simulink model "Simulador_lineal"  (R2023a)
settings: Solver=FixedStepAuto  StartTime=0.0  StopTime=70  FixedStep=Ts  RelTol=1e-3
undefined symbols (not defined in the file): FC, NP, Ts, TsMot, TsPos, TsRef, TsSenF, TsVel, uo
libraries: simulink x1
settings Model: Creator=rrico  LastModifiedBy=jarico
settings OptimizationCC: ReuseModelBlockBuffer=off

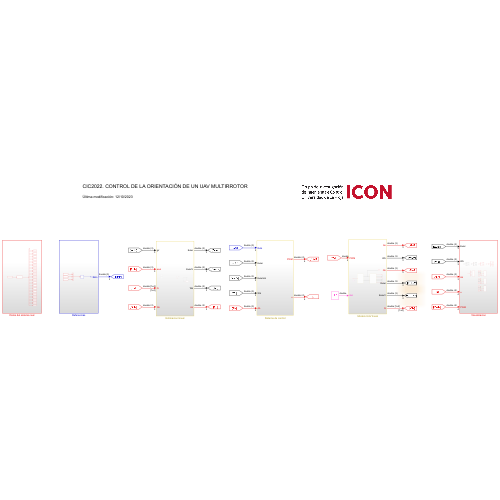
[thumbnail: Simulink's stored preview of the top-level diagram]
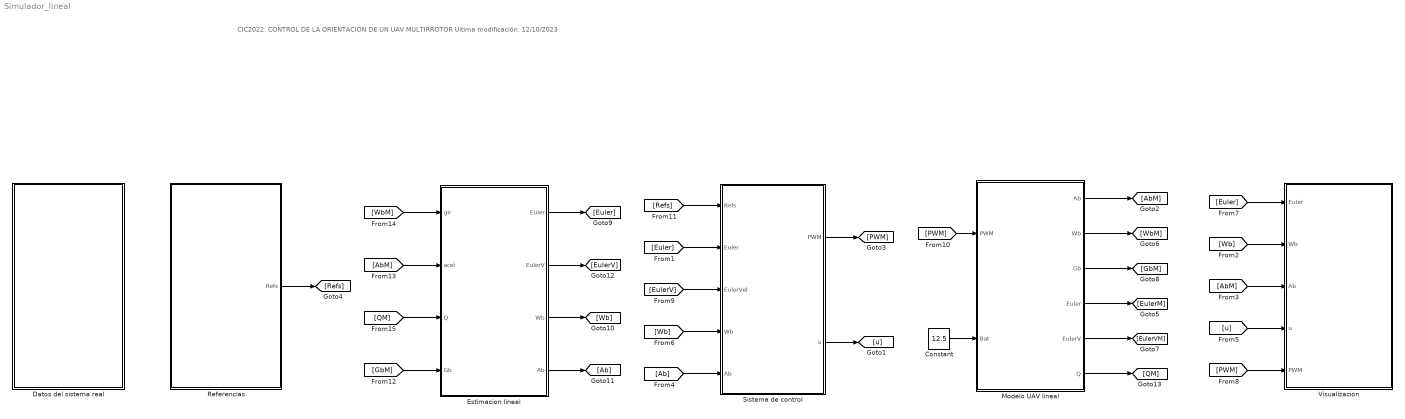
== system Simulador_lineal ==
  note: CIC2022. CONTROL DE LA ORIENTACIÓN DE UN UAV MULTIRROTOR
      |
      | Última modificación: 12/10/2023
  Constant : Constant  Value=12.5
  Datos del sistema real : Subsystem
  Estimacion lineal : Subsystem
  Modelo UAV lineal : Subsystem
  Referencias : Subsystem
  Sistema de control : Subsystem
  Visualizacion : Subsystem
  wires:
  Referencias/1(Refs) -> [Refs]
  [Wb] -> Visualizacion/2(Wb)
  [AbM] -> Visualizacion/3(Ab)
  [PWM] -> Visualizacion/5(PWM)
  [u] -> Visualizacion/4(u)
  Constant/1 -> Modelo UAV lineal/2(Bat)
  Sistema de control/1(PWM) -> [PWM]
  [PWM] -> Modelo UAV lineal/1(PWM)
  Modelo UAV lineal/2(Wb) -> [WbM]
  Modelo UAV lineal/1(Ab) -> [AbM]
  [Refs] -> Sistema de control/1(Refs)
  [Wb] -> Sistema de control/4(Wb)
  Sistema de control/2(u) -> [u]
  [Euler] -> Sistema de control/2(Euler)
  Modelo UAV lineal/4(Euler) -> [EulerM]
  [Euler] -> Visualizacion/1(Euler)
  [Ab] -> Sistema de control/5(Ab)
  Modelo UAV lineal/5(EulerV) -> [EulerVM]
  [EulerV] -> Sistema de control/3(EulerVel)
  Modelo UAV lineal/3(Gb) -> [GbM]
  Estimacion lineal/1(Euler) -> [Euler]
  Estimacion lineal/3(Wb) -> [Wb]
  Estimacion lineal/4(Ab) -> [Ab]
  Estimacion lineal/2(EulerV) -> [EulerV]
  Modelo UAV lineal/6(Q) -> [QM]
  [GbM] -> Estimacion lineal/4(Gb)
  [QM] -> Estimacion lineal/3(Q)
  [AbM] -> Estimacion lineal/2(acel)
  [WbM] -> Estimacion lineal/1(gir)

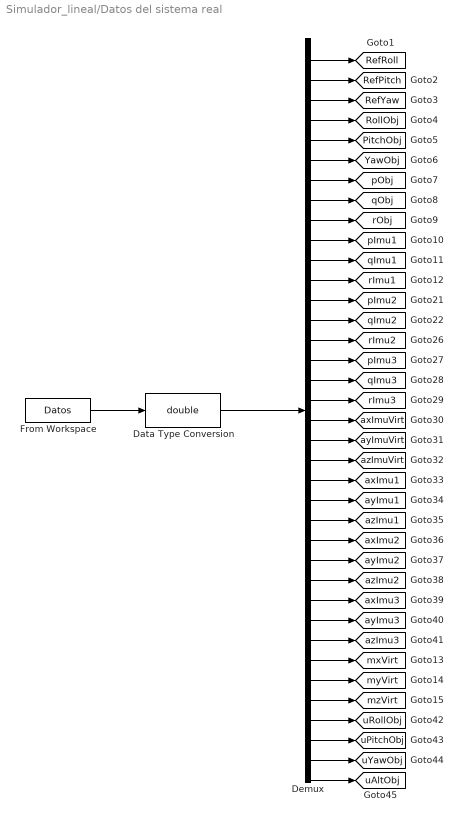
== system Simulador_lineal/Datos del sistema real ==
  Data Type Conversion : DataTypeConversion  OutDataTypeStr=double  SaturateOnIntegerOverflow=off  RndMeth=Floor
  Demux : Demux  Outputs=38
  From Workspace : FromWorkspace  VariableName=Datos  SampleTime=Ts
  tag scope: PitchObj=global, RefPitch=global, RefRoll=global, RefYaw=global, RollObj=global, YawObj=global, axImu1=global, axImu2=global, axImu3=global, axImuVirt=global, ayImu1=global, ayImu2=global, ayImu3=global, ayImuVirt=global, azImu1=global, azImu2=global, azImu3=global, azImuVirt=global, mxVirt=global, myVirt=global, mzVirt=global, pImu1=global, pImu2=global, pImu3=global, pObj=global, qImu1=global, qImu2=global, qImu3=global, qObj=global, rImu1=global, rImu2=global, rImu3=global, rObj=global, uAltObj=global, uPitchObj=global, uRollObj=global, uYawObj=global
  wires:
  Demux/31 -> [azImu3]
  Demux/7 -> [YawObj]
  Demux/17 -> [pImu3]
  Demux/25 -> [azImu1]
  Demux/27 -> [ayImu2]
  Demux/16 -> [rImu2]
  Demux/15 -> [qImu2]
  Demux/30 -> [ayImu3]
  Demux/21 -> [ayImuVirt]
  Demux/10 -> [rObj]
  Demux/2 -> [RefRoll]
  Demux/24 -> [ayImu1]
  Demux/5 -> [RollObj]
  Demux/29 -> [axImu3]
  Demux/8 -> [pObj]
  Demux/28 -> [azImu2]
  Demux/18 -> [qImu3]
  Demux/6 -> [PitchObj]
  Demux/19 -> [rImu3]
  Data Type Conversion/1 -> Demux/1
  Demux/4 -> [RefYaw]
  Demux/22 -> [azImuVirt]
  From Workspace/1 -> Data Type Conversion/1
  Demux/23 -> [axImu1]
  Demux/9 -> [qObj]
  Demux/13 -> [rImu1]
  Demux/3 -> [RefPitch]
  Demux/26 -> [axImu2]
  Demux/11 -> [pImu1]
  Demux/14 -> [pImu2]
  Demux/38 -> [uAltObj]
  Demux/37 -> [uYawObj]
  Demux/36 -> [uPitchObj]
  Demux/35 -> [uRollObj]
  Demux/32 -> [mxVirt]
  Demux/33 -> [myVirt]
  Demux/34 -> [mzVirt]
  Demux/20 -> [axImuVirt]
  Demux/12 -> [qImu1]

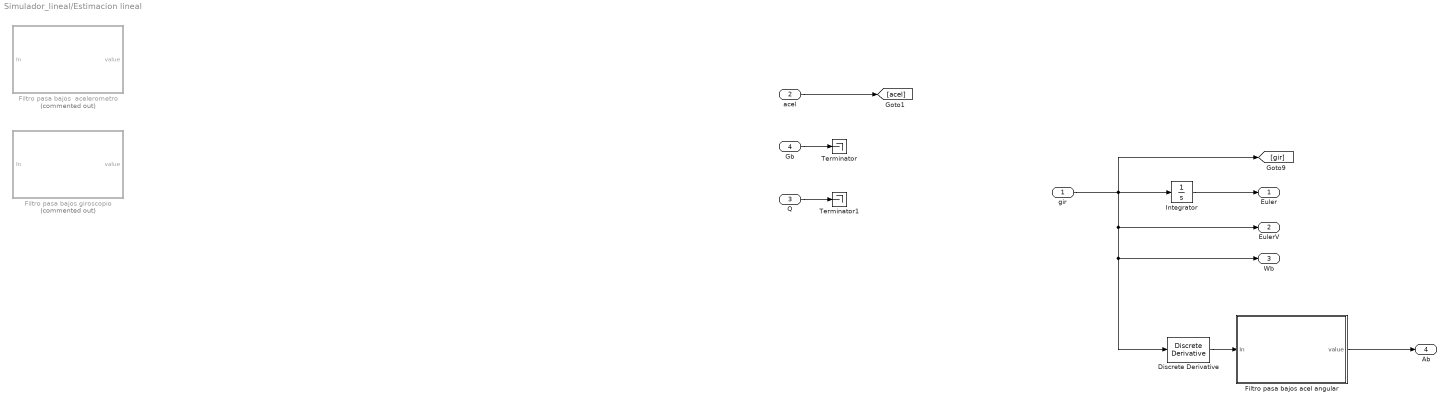
== system Simulador_lineal/Estimacion lineal ==
  gir : Inport
  acel : Inport  Port=2
  Q : Inport  Port=3
  Gb : Inport  Port=4
  Discrete Derivative : simulink/Discrete/Discrete Derivative  gainval=1.0  ICPrevScaledInput=0.0  OutMin=[]  OutMax=[]  OutDataType=fixdt(1, 16)  OutScaling=2^-10  DoSatur=off
  Filtro pasa bajos  acelerometro : Subsystem  Commented=on  TreatAsAtomicUnit=on  SystemSampleTime=TsSenF  mask{P=NP, Fc=FC, TsF=TsSenF}
      mask prompts: P "Polos"; Fc "Frecuencia de corte"; TsF "Tiempo de muestreo"
      mask DialogControl ParameterGroup1 Prompt: Parameters
  Filtro pasa bajos acel angular : Subsystem  TreatAsAtomicUnit=on  SystemSampleTime=TsVel  mask{P=2, Fc=30, TsF=TsSenF}
      mask prompts: P "Polos"; Fc "Frecuencia de corte"; TsF "Tiempo de muestreo"
      mask DialogControl ParameterGroup1 Prompt: Parameters
  Filtro pasa bajos giroscopio : Subsystem  Commented=on  TreatAsAtomicUnit=on  SystemSampleTime=TsSenF  mask{P=NP, Fc=FC, TsF=TsSenF}
      mask prompts: P "Polos"; Fc "Frecuencia de corte"; TsF "Tiempo de muestreo"
      mask DialogControl ParameterGroup1 Prompt: Parameters
  Integrator : Integrator
  Terminator : Terminator
  Terminator1 : Terminator
  Euler : Outport
  EulerV : Outport  Port=2
  Wb : Outport  Port=3
  Ab : Outport  Port=4
  wires:
  Discrete Derivative/1 -> Filtro pasa bajos acel angular/1(In)
  Filtro pasa bajos acel angular/1(value) -> Ab/1
  Gb/1 -> Terminator/1
  Q/1 -> Terminator1/1
  acel/1 -> [acel]
  gir/1 -> [gir], Integrator/1, Discrete Derivative/1, Wb/1, EulerV/1
  Integrator/1 -> Euler/1

== system Simulador_lineal/Modelo UAV lineal ==
  PWM : Inport
  Bat : Inport  Port=2
  Dinamica UAV : Subsystem  mask{Mo=[0 0 0], B=[0.002 0.005 0.005]*0, F=[0.025 0.006 0.006]*0, I=[0.0014 0.025 0.0549], Im=0.0005, dM=0, M=0.2472, Dr=0.09, Dp=0.0675, Y=off, Mq=on}
      mask prompts: Mo "Par inicial"; B "Rozamiento viscoso"; F "Rozamiento estático"; I "Inercia"; Im "Inercia del rotor"; dM "Distancia del centro de masas"; M "Masa"; Dr "Distancia de los rotores a roll"; Dp "Distancia de los rotores a pitch"; Y "Habilitacion yaw"; Mq "Modelo de maqueta"
      mask DialogControl DescTextVar Prompt: Modelo dinámico del UAV
      mask DialogControl Parameter1 Prompt: Rozamientos y pares adicionales
      mask DialogControl Parameter2 Prompt: Parámetros físicos
      mask DialogControl Parameter3 Prompt: Selectores
  Scope : Scope
  Sistema de propulsion : Subsystem  mask{k=9.0893, kd=0, Tau=0.05}
      mask prompts: k "Ganancia en thrust"; kd "Ganancia en drag"; Tau "Dinamica"
      mask DialogControl ParameterGroupVar1 Prompt: Estatica del motor
      mask DialogControl ParameterGroupVar2 Prompt: Dinamica del motor
  Terminator : Terminator
  Ab : Outport
  Wb : Outport  Port=2
  Gb : Outport  Port=3
  Euler : Outport  Port=4
  EulerV : Outport  Port=5
  Q : Outport  Port=6
  wires:
  Dinamica UAV/6(Q) -> Q/1
  Dinamica UAV/5(EulerV) -> EulerV/1
  Dinamica UAV/4(Euler) -> Euler/1
  Dinamica UAV/1(Ab) -> Ab/1
  Sistema de propulsion/1(T) -> Scope/1, Dinamica UAV/1(T)
  Dinamica UAV/2(Wb) -> Wb/1
  Sistema de propulsion/2(D) -> Dinamica UAV/2(Delta)
  Dinamica UAV/3(Gb) -> Gb/1
  PWM/1 -> Sistema de propulsion/1(PWM)
  Bat/1 -> Terminator/1

== system Simulador_lineal/Referencias ==
  Mux17 : Mux  Inputs=3
  Zero-Order Hold : ZeroOrderHold  SampleTime=TsRef
  Refs : Outport  VectorParamsAs1DForOutWhenUnconnected=off
  wires:
  Zero-Order Hold/1 -> Refs/1
  [RefYaw] -> Mux17/3
  [RefPitch] -> Mux17/2
  [RefRoll] -> Mux17/1
  Mux17/1 -> Zero-Order Hold/1

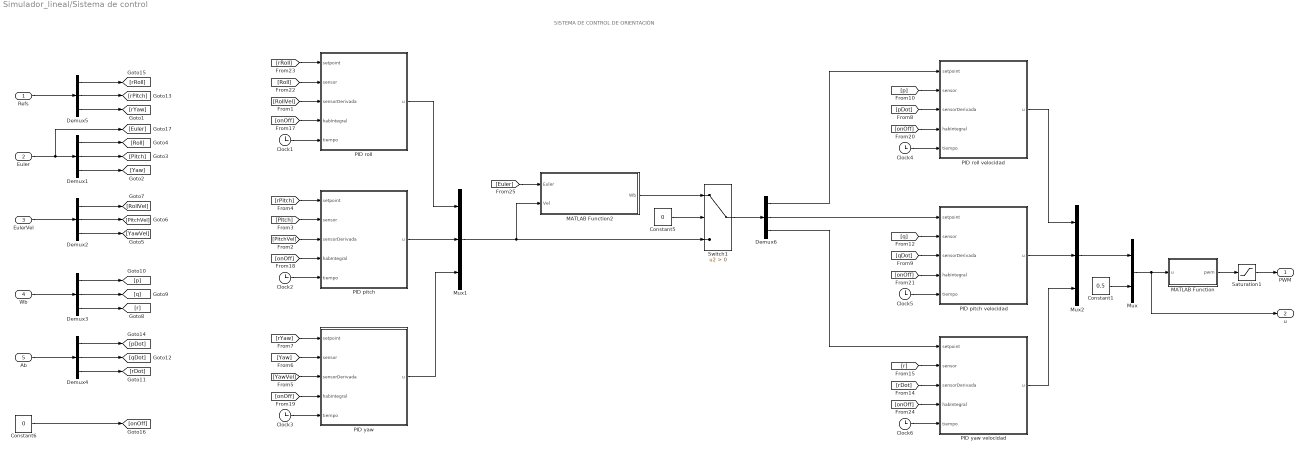
== system Simulador_lineal/Sistema de control ==
  note: SISTEMA DE CONTROL DE ORIENTACIÓN
  Refs : Inport
  Euler : Inport  Port=2
  EulerVel : Inport  Port=3
  Wb : Inport  Port=4
  Ab : Inport  Port=5
  Clock{1..6} (6 alike) : Clock
  Constant1 : Constant  Value=0.5  SampleTime=-1
  Constant5 : Constant  Value=0
  Constant6 : Constant  Value=0  SampleTime=-1
  Demux{1..6} (6 alike) : Demux  Outputs=3
  MATLAB Function : MATLAB Function  TreatAsAtomicUnit=on
  MATLAB Function2 : MATLAB Function  TreatAsAtomicUnit=on  SystemSampleTime=TsVel
  Mux : Mux  Inputs=2
  Mux1 : Mux  Inputs=3
  Mux2 : Mux  Inputs=3
  PID pitch : Subsystem  TreatAsAtomicUnit=on  SystemSampleTime=TsPos  mask{Kp=4, Ki=0, Kd=0, Kff=0, LimI=2000, LimT=2000}
      mask prompts: LimI "Limite I"; LimT "Limite total"
  PID pitch velocidad : Subsystem  TreatAsAtomicUnit=on  SystemSampleTime=TsVel  mask{Kp=0.0024, Ki=0.000378, Kd=0, Kff=0, LimI=1, LimT=1}
      mask prompts: LimI "Limite I"; LimT "Limite total"
  PID roll : Subsystem  TreatAsAtomicUnit=on  SystemSampleTime=TsPos  mask{Kp=5, Ki=0, Kd=0, Kff=0, LimI=2000, LimT=2000}
      mask prompts: LimI "Limite I"; LimT "Limite total"
  PID roll velocidad : Subsystem  TreatAsAtomicUnit=on  SystemSampleTime=TsVel  mask{Kp=0.00051, Ki=0.000000153, Kd=0, Kff=0, LimI=1, LimT=1}
      mask prompts: LimI "Limite I"; LimT "Limite total"
  PID yaw : Subsystem  TreatAsAtomicUnit=on  SystemSampleTime=TsPos  mask{Kp=0, Ki=0, Kd=0, Kff=0, LimI=2000, LimT=2000}
      mask prompts: LimI "Limite I"; LimT "Limite total"
  PID yaw velocidad : Subsystem  TreatAsAtomicUnit=on  SystemSampleTime=TsVel  mask{Kp=0, Ki=0, Kd=0, Kff=0, LimI=1, LimT=1}
      mask prompts: LimI "Limite I"; LimT "Limite total"
  Saturation1 : Saturate  UpperLimit=1  LowerLimit=0
  Switch1 : Switch  Criteria=u2 > Threshold  SaturateOnIntegerOverflow=off  InputSameDT=off
  PWM : Outport  VectorParamsAs1DForOutWhenUnconnected=off
  u : Outport  Port=2  VectorParamsAs1DForOutWhenUnconnected=off
  wires:
  Saturation1/1 -> PWM/1
  MATLAB Function/1(pwm) -> Saturation1/1
  Constant1/1 -> Mux/2
  Mux/1 -> u/1, MATLAB Function/1(u)
  [Pitch] -> PID pitch/2(sensor)
  [rPitch] -> PID pitch/1(setpoint)
  [Yaw] -> PID yaw/2(sensor)
  [YawVel] -> PID yaw/3(sensorDerivada)
  [Roll] -> PID roll/2(sensor)
  [RollVel] -> PID roll/3(sensorDerivada)
  [rYaw] -> PID yaw/1(setpoint)
  [rRoll] -> PID roll/1(setpoint)
  PID pitch/1(u) -> Mux1/2
  [onOff] -> PID roll/4(habIntegral)
  PID yaw/1(u) -> Mux1/3
  [PitchVel] -> PID pitch/3(sensorDerivada)
  PID roll/1(u) -> Mux1/1
  PID pitch velocidad/1(u) -> Mux2/2
  PID roll velocidad/1(u) -> Mux2/1
  [p] -> PID roll velocidad/2(sensor)
  Demux6/1 -> PID roll velocidad/1(setpoint)
  [r] -> PID yaw velocidad/2(sensor)
  [pDot] -> PID roll velocidad/3(sensorDerivada)
  Demux6/3 -> PID yaw velocidad/1(setpoint)
  PID yaw velocidad/1(u) -> Mux2/3
  Demux6/2 -> PID pitch velocidad/1(setpoint)
  [qDot] -> PID pitch velocidad/3(sensorDerivada)
  Mux2/1 -> Mux/1
  [q] -> PID pitch velocidad/2(sensor)
  [rDot] -> PID yaw velocidad/3(sensorDerivada)
  Demux1/2 -> [Pitch]
  Demux2/1 -> [RollVel]
  Demux5/1 -> [rRoll]
  Demux5/3 -> [rYaw]
  Demux2/3 -> [YawVel]
  Demux1/3 -> [Yaw]
  Demux1/1 -> [Roll]
  Demux2/2 -> [PitchVel]
  Demux5/2 -> [rPitch]
  Demux3/2 -> [q]
  Demux3/1 -> [p]
  Demux4/3 -> [rDot]
  Demux3/3 -> [r]
  Demux4/1 -> [pDot]
  Demux4/2 -> [qDot]
  Constant6/1 -> [onOff]
  [onOff] -> PID pitch/4(habIntegral)
  Clock1/1 -> PID roll/5(tiempo)
  [onOff] -> PID yaw/4(habIntegral)
  [onOff] -> PID roll velocidad/4(habIntegral)
  [onOff] -> PID pitch velocidad/4(habIntegral)
  [onOff] -> PID yaw velocidad/4(habIntegral)
  Constant5/1 -> Switch1/2
  MATLAB Function2/1(Wb) -> Switch1/1
  Mux1/1 -> MATLAB Function2/2(Vel), Switch1/3
  [Euler] -> MATLAB Function2/1(Euler)
  Switch1/1 -> Demux6/1
  Ab/1 -> Demux4/1
  Wb/1 -> Demux3/1
  EulerVel/1 -> Demux2/1
  Euler/1 -> [Euler], Demux1/1
  Refs/1 -> Demux5/1
  Clock2/1 -> PID pitch/5(tiempo)
  Clock3/1 -> PID yaw/5(tiempo)
  Clock4/1 -> PID roll velocidad/5(tiempo)
  Clock5/1 -> PID pitch velocidad/5(tiempo)
  Clock6/1 -> PID yaw velocidad/5(tiempo)

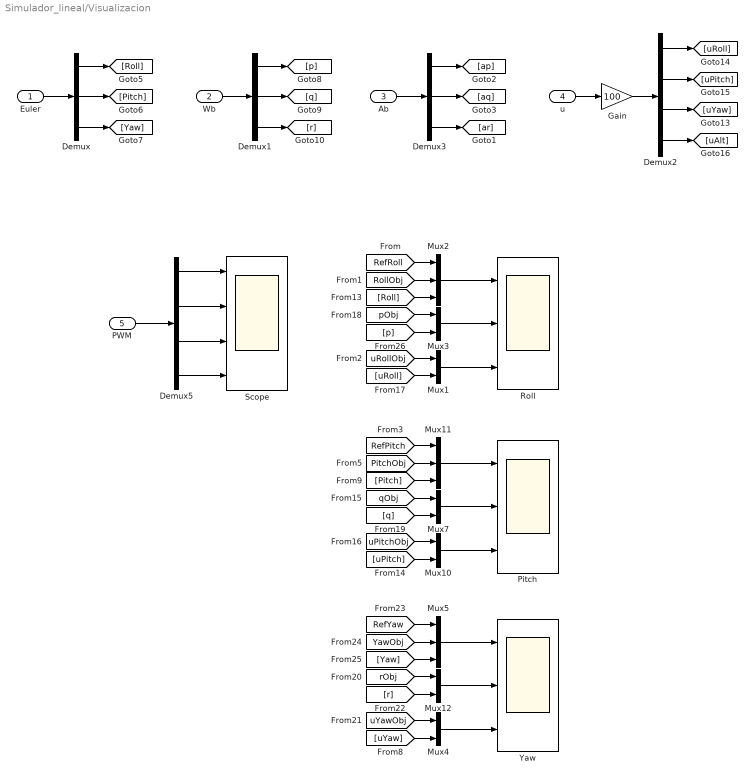
== system Simulador_lineal/Visualizacion ==
  Euler : Inport
  Wb : Inport  Port=2
  Ab : Inport  Port=3
  u : Inport  Port=4
  PWM : Inport  Port=5
  Demux : Demux  Outputs=3
  Demux1 : Demux  Outputs=3
  Demux2 : Demux
  Demux3 : Demux  Outputs=3
  Demux5 : Demux
  Gain : Gain  Gain=100
  Mux{1,3..4,7,10,12} (6 alike) : Mux  Inputs=2
  Mux11 : Mux  Inputs=3
  Mux2 : Mux  Inputs=3
  Mux5 : Mux  Inputs=3
  Pitch : Scope  NumInputPorts=3
  Roll : Scope  NumInputPorts=3
  Scope : Scope  NumInputPorts=4
  Yaw : Scope  NumInputPorts=3
  wires:
  [YawObj] -> Mux5/2
  [r] -> Mux12/2
  Mux11/1 -> Pitch/1
  [uYawObj] -> Mux4/1
  Demux/3 -> [Yaw]
  [uPitchObj] -> Mux10/1
  [RefYaw] -> Mux5/1
  Demux1/2 -> [q]
  Euler/1 -> Demux/1
  [Yaw] -> Mux5/3
  Demux/2 -> [Pitch]
  [rObj] -> Mux12/1
  Demux1/1 -> [p]
  [q] -> Mux7/2
  Wb/1 -> Demux1/1
  Demux1/3 -> [r]
  [qObj] -> Mux7/1
  Demux/1 -> [Roll]
  [uYaw] -> Mux4/2
  Demux2/3 -> [uYaw]
  Demux2/2 -> [uPitch]
  Demux2/1 -> [uRoll]
  u/1 -> Gain/1
  [PitchObj] -> Mux11/2
  [RefPitch] -> Mux11/1
  [Pitch] -> Mux11/3
  Demux2/4 -> [uAlt]
  Mux10/1 -> Pitch/3
  Mux7/1 -> Pitch/2
  [uPitch] -> Mux10/2
  Mux5/1 -> Yaw/1
  Mux12/1 -> Yaw/2
  Mux4/1 -> Yaw/3
  Demux3/3 -> [ar]
  Ab/1 -> Demux3/1
  Demux3/1 -> [ap]
  Demux3/2 -> [aq]
  Gain/1 -> Demux2/1
  PWM/1 -> Demux5/1
  Demux5/1 -> Scope/1
  Demux5/3 -> Scope/3
  Demux5/2 -> Scope/2
  Demux5/4 -> Scope/4
  [uRoll] -> Mux1/2
  [Roll] -> Mux2/3
  Mux2/1 -> Roll/1
  Mux1/1 -> Roll/3
  [RollObj] -> Mux2/2
  [pObj] -> Mux3/1
  [p] -> Mux3/2
  Mux3/1 -> Roll/2
  [RefRoll] -> Mux2/1
  [uRollObj] -> Mux1/1

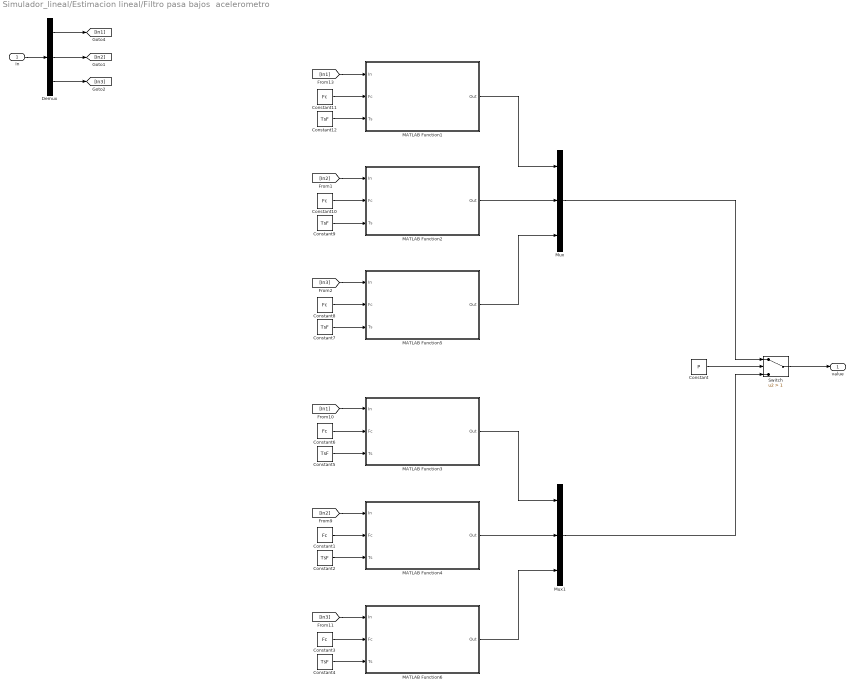
== system Simulador_lineal/Estimacion lineal/Filtro pasa bajos  acelerometro ==
  In : Inport
  Constant : Constant  Value=P
  Constant{1,3,6,8,10..11} (6 alike) : Constant  Value=Fc
  Constant{2,4..5,7,9,12} (6 alike) : Constant  Value=TsF
  Demux : Demux  Outputs=3
  MATLAB Function1 : MATLAB Function  TreatAsAtomicUnit=on
  MATLAB Function2 : MATLAB Function  TreatAsAtomicUnit=on
  MATLAB Function3 : MATLAB Function  TreatAsAtomicUnit=on
  MATLAB Function4 : MATLAB Function  TreatAsAtomicUnit=on
  MATLAB Function5 : MATLAB Function  TreatAsAtomicUnit=on
  MATLAB Function6 : MATLAB Function  TreatAsAtomicUnit=on
  Mux : Mux  Inputs=3
  Mux1 : Mux  Inputs=3
  Switch : Switch  Criteria=u2 > Threshold  Threshold=1  SaturateOnIntegerOverflow=off  InputSameDT=off
  value : Outport
  wires:
  Constant/1 -> Switch/2
  Switch/1 -> value/1
  [In1] -> MATLAB Function1/1(In)
  MATLAB Function2/1(Out) -> Mux/2
  MATLAB Function1/1(Out) -> Mux/1
  MATLAB Function5/1(Out) -> Mux/3
  Mux/1 -> Switch/1
  In/1 -> Demux/1
  Demux/1 -> [In1]
  Demux/2 -> [In2]
  Demux/3 -> [In3]
  [In2] -> MATLAB Function2/1(In)
  [In3] -> MATLAB Function5/1(In)
  Constant4/1 -> MATLAB Function6/3(Ts)
  Constant3/1 -> MATLAB Function6/2(Fc)
  Constant1/1 -> MATLAB Function4/2(Fc)
  Constant2/1 -> MATLAB Function4/3(Ts)
  [In3] -> MATLAB Function6/1(In)
  [In2] -> MATLAB Function4/1(In)
  [In1] -> MATLAB Function3/1(In)
  MATLAB Function3/1(Out) -> Mux1/1
  MATLAB Function4/1(Out) -> Mux1/2
  MATLAB Function6/1(Out) -> Mux1/3
  Mux1/1 -> Switch/3
  Constant5/1 -> MATLAB Function3/3(Ts)
  Constant6/1 -> MATLAB Function3/2(Fc)
  Constant7/1 -> MATLAB Function5/3(Ts)
  Constant8/1 -> MATLAB Function5/2(Fc)
  Constant10/1 -> MATLAB Function2/2(Fc)
  Constant9/1 -> MATLAB Function2/3(Ts)
  Constant12/1 -> MATLAB Function1/3(Ts)
  Constant11/1 -> MATLAB Function1/2(Fc)

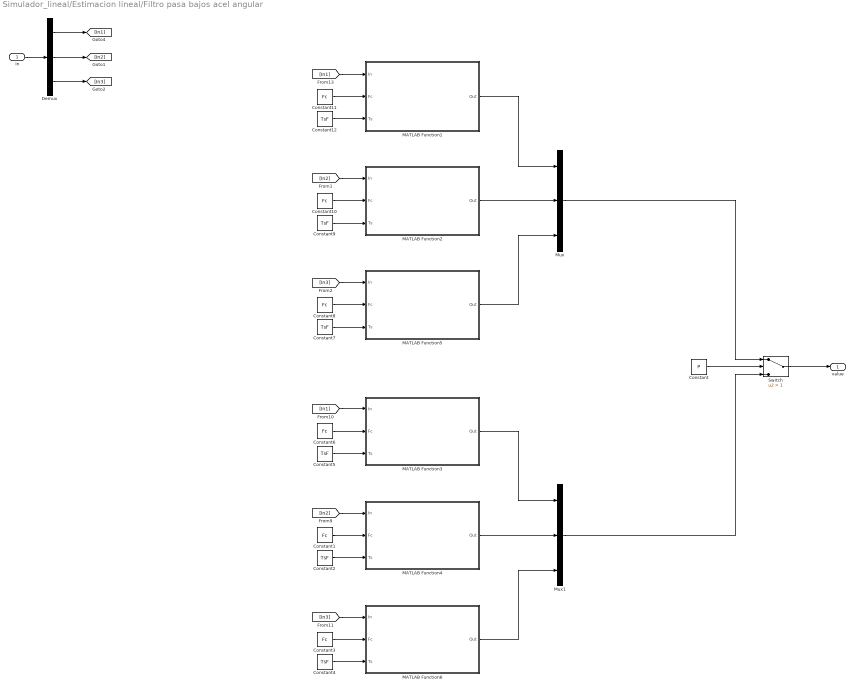
== system Simulador_lineal/Estimacion lineal/Filtro pasa bajos acel angular ==
  In : Inport
  Constant : Constant  Value=P
  Constant{1,3,6,8,10..11} (6 alike) : Constant  Value=Fc
  Constant{2,4..5,7,9,12} (6 alike) : Constant  Value=TsF
  Demux : Demux  Outputs=3
  MATLAB Function1 : MATLAB Function  TreatAsAtomicUnit=on
  MATLAB Function2 : MATLAB Function  TreatAsAtomicUnit=on
  MATLAB Function3 : MATLAB Function  TreatAsAtomicUnit=on
  MATLAB Function4 : MATLAB Function  TreatAsAtomicUnit=on
  MATLAB Function5 : MATLAB Function  TreatAsAtomicUnit=on
  MATLAB Function6 : MATLAB Function  TreatAsAtomicUnit=on
  Mux : Mux  Inputs=3
  Mux1 : Mux  Inputs=3
  Switch : Switch  Criteria=u2 > Threshold  Threshold=1  SaturateOnIntegerOverflow=off  InputSameDT=off
  value : Outport
  wires:
  Constant/1 -> Switch/2
  Switch/1 -> value/1
  [In1] -> MATLAB Function1/1(In)
  MATLAB Function2/1(Out) -> Mux/2
  MATLAB Function1/1(Out) -> Mux/1
  MATLAB Function5/1(Out) -> Mux/3
  Mux/1 -> Switch/1
  In/1 -> Demux/1
  Demux/1 -> [In1]
  Demux/2 -> [In2]
  Demux/3 -> [In3]
  [In2] -> MATLAB Function2/1(In)
  [In3] -> MATLAB Function5/1(In)
  Constant4/1 -> MATLAB Function6/3(Ts)
  Constant3/1 -> MATLAB Function6/2(Fc)
  Constant1/1 -> MATLAB Function4/2(Fc)
  Constant2/1 -> MATLAB Function4/3(Ts)
  [In3] -> MATLAB Function6/1(In)
  [In2] -> MATLAB Function4/1(In)
  [In1] -> MATLAB Function3/1(In)
  MATLAB Function3/1(Out) -> Mux1/1
  MATLAB Function4/1(Out) -> Mux1/2
  MATLAB Function6/1(Out) -> Mux1/3
  Mux1/1 -> Switch/3
  Constant5/1 -> MATLAB Function3/3(Ts)
  Constant6/1 -> MATLAB Function3/2(Fc)
  Constant7/1 -> MATLAB Function5/3(Ts)
  Constant8/1 -> MATLAB Function5/2(Fc)
  Constant10/1 -> MATLAB Function2/2(Fc)
  Constant9/1 -> MATLAB Function2/3(Ts)
  Constant12/1 -> MATLAB Function1/3(Ts)
  Constant11/1 -> MATLAB Function1/2(Fc)

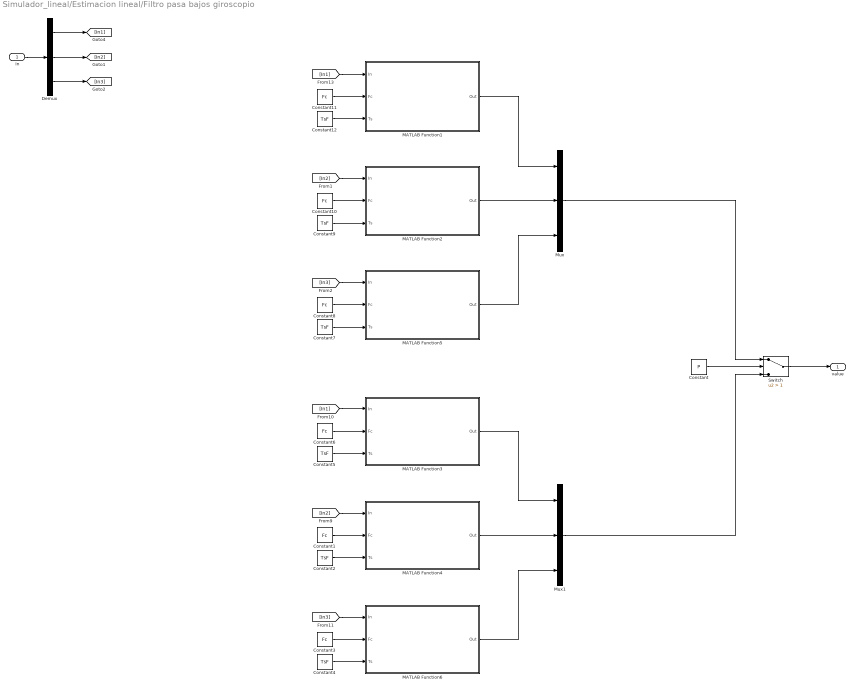
== system Simulador_lineal/Estimacion lineal/Filtro pasa bajos giroscopio ==
  In : Inport
  Constant : Constant  Value=P
  Constant{1,3,6,8,10..11} (6 alike) : Constant  Value=Fc
  Constant{2,4..5,7,9,12} (6 alike) : Constant  Value=TsF
  Demux : Demux  Outputs=3
  MATLAB Function1 : MATLAB Function  TreatAsAtomicUnit=on
  MATLAB Function2 : MATLAB Function  TreatAsAtomicUnit=on
  MATLAB Function3 : MATLAB Function  TreatAsAtomicUnit=on
  MATLAB Function4 : MATLAB Function  TreatAsAtomicUnit=on
  MATLAB Function5 : MATLAB Function  TreatAsAtomicUnit=on
  MATLAB Function6 : MATLAB Function  TreatAsAtomicUnit=on
  Mux : Mux  Inputs=3
  Mux1 : Mux  Inputs=3
  Switch : Switch  Criteria=u2 > Threshold  Threshold=1  SaturateOnIntegerOverflow=off  InputSameDT=off
  value : Outport
  wires:
  Constant11/1 -> MATLAB Function1/2(Fc)
  Constant12/1 -> MATLAB Function1/3(Ts)
  Constant9/1 -> MATLAB Function2/3(Ts)
  Constant10/1 -> MATLAB Function2/2(Fc)
  Constant8/1 -> MATLAB Function5/2(Fc)
  Constant7/1 -> MATLAB Function5/3(Ts)
  Constant6/1 -> MATLAB Function3/2(Fc)
  Constant5/1 -> MATLAB Function3/3(Ts)
  Mux1/1 -> Switch/3
  MATLAB Function6/1(Out) -> Mux1/3
  MATLAB Function4/1(Out) -> Mux1/2
  MATLAB Function3/1(Out) -> Mux1/1
  [In1] -> MATLAB Function3/1(In)
  [In2] -> MATLAB Function4/1(In)
  [In3] -> MATLAB Function6/1(In)
  Constant2/1 -> MATLAB Function4/3(Ts)
  Constant1/1 -> MATLAB Function4/2(Fc)
  Constant3/1 -> MATLAB Function6/2(Fc)
  Constant4/1 -> MATLAB Function6/3(Ts)
  [In3] -> MATLAB Function5/1(In)
  [In2] -> MATLAB Function2/1(In)
  Demux/3 -> [In3]
  Demux/2 -> [In2]
  Demux/1 -> [In1]
  In/1 -> Demux/1
  Mux/1 -> Switch/1
  MATLAB Function5/1(Out) -> Mux/3
  MATLAB Function1/1(Out) -> Mux/1
  MATLAB Function2/1(Out) -> Mux/2
  [In1] -> MATLAB Function1/1(In)
  Switch/1 -> value/1
  Constant/1 -> Switch/2

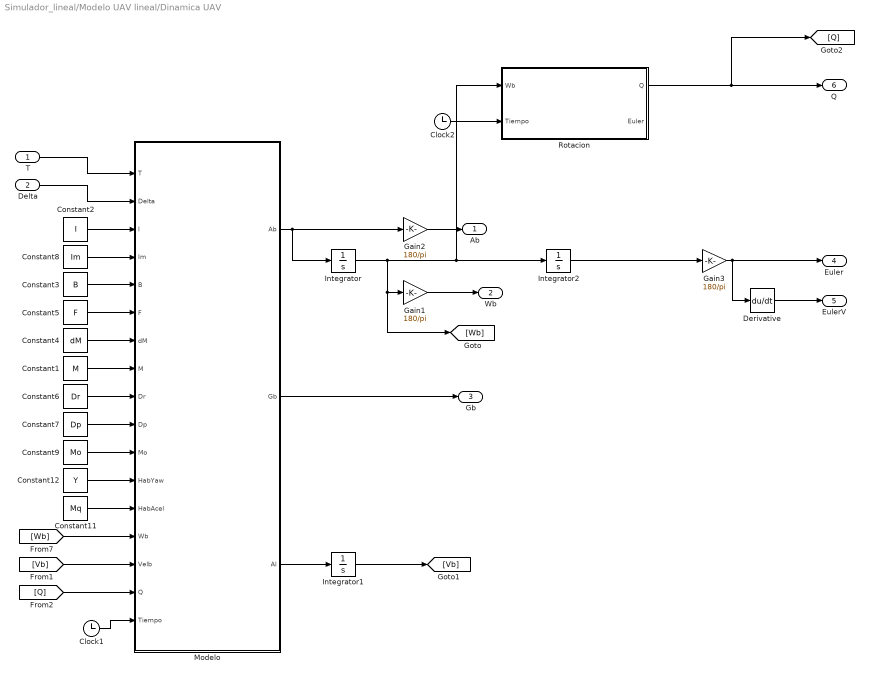
== system Simulador_lineal/Modelo UAV lineal/Dinamica UAV ==
  T : Inport
  Delta : Inport  Port=2
  Clock1 : Clock
  Clock2 : Clock
  Constant1 : Constant  Value=M
  Constant11 : Constant  Value=Mq
  Constant12 : Constant  Value=Y
  Constant2 : Constant  Value=I
  Constant3 : Constant  Value=B
  Constant4 : Constant  Value=dM
  Constant5 : Constant  Value=F
  Constant6 : Constant  Value=Dr
  Constant7 : Constant  Value=Dp
  Constant8 : Constant  Value=Im
  Constant9 : Constant  Value=Mo
  Derivative : Derivative
  Gain1 : Gain  Gain=180/pi
  Gain2 : Gain  Gain=180/pi
  Gain3 : Gain  Gain=180/pi
  Integrator : Integrator
  Integrator1 : Integrator
  Integrator2 : Integrator
  Modelo : MATLAB Function
  Rotacion : MATLAB Function
  Ab : Outport  VectorParamsAs1DForOutWhenUnconnected=off
  Wb : Outport  Port=2  VectorParamsAs1DForOutWhenUnconnected=off
  Gb : Outport  Port=3  VectorParamsAs1DForOutWhenUnconnected=off
  Euler : Outport  Port=4  VectorParamsAs1DForOutWhenUnconnected=off
  EulerV : Outport  Port=5  VectorParamsAs1DForOutWhenUnconnected=off
  Q : Outport  Port=6  VectorParamsAs1DForOutWhenUnconnected=off
  wires:
  Modelo/3(Al) -> Integrator1/1
  Constant11/1 -> Modelo/13(HabAcel)
  Integrator2/1 -> Gain3/1
  [Q] -> Modelo/16(Q)
  Rotacion/1(Q) -> [Q], Q/1
  [Vb] -> Modelo/15(Velb)
  Integrator1/1 -> [Vb]
  Clock1/1 -> Modelo/17(Tiempo)
  Derivative/1 -> EulerV/1
  Gain3/1 -> Derivative/1, Euler/1
  [Wb] -> Modelo/14(Wb)
  Clock2/1 -> Rotacion/2(Tiempo)
  Constant12/1 -> Modelo/12(HabYaw)
  Gain2/1 -> Ab/1
  Gain1/1 -> Wb/1
  Constant7/1 -> Modelo/10(Dp)
  Modelo/1(Ab) -> Gain2/1, Integrator/1
  Integrator/1 -> Rotacion/1(Wb), Integrator2/1, [Wb], Gain1/1
  Constant5/1 -> Modelo/6(F)
  Constant2/1 -> Modelo/3(I)
  Modelo/2(Gb) -> Gb/1
  Constant9/1 -> Modelo/11(Mo)
  Constant1/1 -> Modelo/8(M)
  Constant3/1 -> Modelo/5(B)
  Constant8/1 -> Modelo/4(Im)
  Constant6/1 -> Modelo/9(Dr)
  Constant4/1 -> Modelo/7(dM)
  T/1 -> Modelo/1(T)
  Delta/1 -> Modelo/2(Delta)

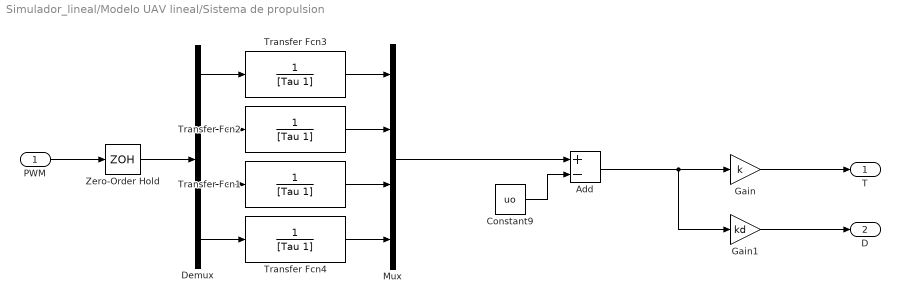
== system Simulador_lineal/Modelo UAV lineal/Sistema de propulsion ==
  PWM : Inport
  Add : Sum  Inputs=+-
  Constant9 : Constant  Value=uo
  Demux : Demux
  Gain : Gain  Gain=k
  Gain1 : Gain  Gain=kd
  Mux : Mux
  Transfer Fcn{1..4} (4 alike) : TransferFcn  Denominator=[Tau 1]
  Zero-Order Hold : ZeroOrderHold  SampleTime=TsMot
  T : Outport
  D : Outport  Port=2
  wires:
  PWM/1 -> Zero-Order Hold/1
  Zero-Order Hold/1 -> Demux/1
  Demux/4 -> Transfer Fcn4/1
  Transfer Fcn4/1 -> Mux/4
  Demux/1 -> Transfer Fcn3/1
  Demux/3 -> Transfer Fcn1/1
  Transfer Fcn1/1 -> Mux/3
  Transfer Fcn2/1 -> Mux/2
  Demux/2 -> Transfer Fcn2/1
  Transfer Fcn3/1 -> Mux/1
  Mux/1 -> Add/1
  Constant9/1 -> Add/2
  Add/1 -> Gain1/1, Gain/1
  Gain/1 -> T/1
  Gain1/1 -> D/1

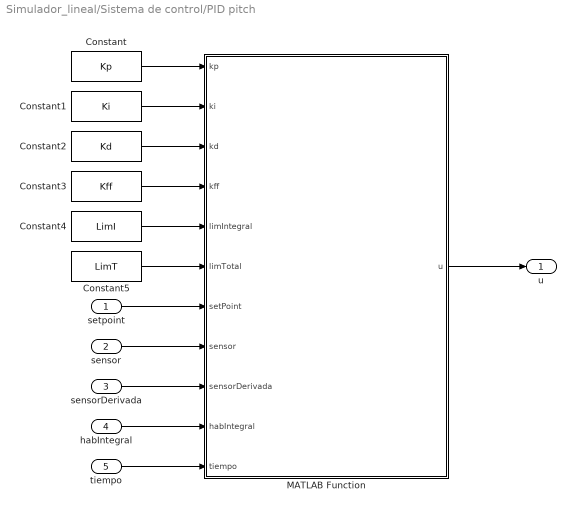
== system Simulador_lineal/Sistema de control/PID pitch ==
  setpoint : Inport
  sensor : Inport  Port=2
  sensorDerivada : Inport  Port=3
  habIntegral : Inport  Port=4
  tiempo : Inport  Port=5
  Constant : Constant  Value=Kp
  Constant1 : Constant  Value=Ki
  Constant2 : Constant  Value=Kd
  Constant3 : Constant  Value=Kff
  Constant4 : Constant  Value=LimI
  Constant5 : Constant  Value=LimT
  MATLAB Function : MATLAB Function  TreatAsAtomicUnit=on
  u : Outport
  wires:
  MATLAB Function/1(u) -> u/1
  tiempo/1 -> MATLAB Function/11(tiempo)
  sensor/1 -> MATLAB Function/8(sensor)
  setpoint/1 -> MATLAB Function/7(setPoint)
  sensorDerivada/1 -> MATLAB Function/9(sensorDerivada)
  Constant1/1 -> MATLAB Function/2(ki)
  Constant3/1 -> MATLAB Function/4(kff)
  Constant4/1 -> MATLAB Function/5(limIntegral)
  Constant5/1 -> MATLAB Function/6(limTotal)
  habIntegral/1 -> MATLAB Function/10(habIntegral)
  Constant2/1 -> MATLAB Function/3(kd)
  Constant/1 -> MATLAB Function/1(kp)

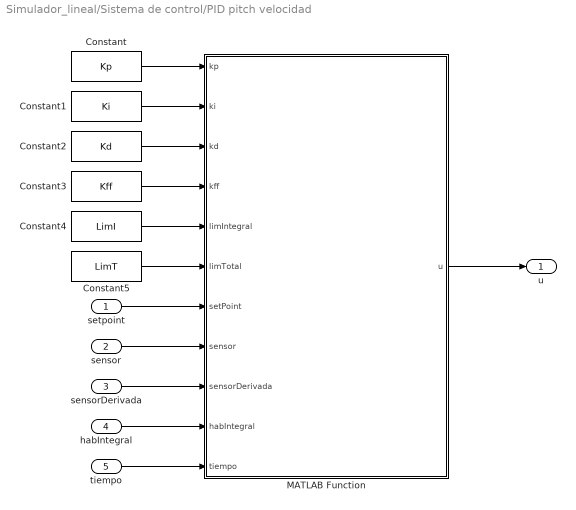
== system Simulador_lineal/Sistema de control/PID pitch velocidad ==
  setpoint : Inport
  sensor : Inport  Port=2
  sensorDerivada : Inport  Port=3
  habIntegral : Inport  Port=4
  tiempo : Inport  Port=5
  Constant : Constant  Value=Kp
  Constant1 : Constant  Value=Ki
  Constant2 : Constant  Value=Kd
  Constant3 : Constant  Value=Kff
  Constant4 : Constant  Value=LimI
  Constant5 : Constant  Value=LimT
  MATLAB Function : MATLAB Function  TreatAsAtomicUnit=on
  u : Outport
  wires:
  Constant/1 -> MATLAB Function/1(kp)
  Constant2/1 -> MATLAB Function/3(kd)
  habIntegral/1 -> MATLAB Function/10(habIntegral)
  Constant5/1 -> MATLAB Function/6(limTotal)
  Constant4/1 -> MATLAB Function/5(limIntegral)
  Constant3/1 -> MATLAB Function/4(kff)
  Constant1/1 -> MATLAB Function/2(ki)
  sensorDerivada/1 -> MATLAB Function/9(sensorDerivada)
  setpoint/1 -> MATLAB Function/7(setPoint)
  sensor/1 -> MATLAB Function/8(sensor)
  tiempo/1 -> MATLAB Function/11(tiempo)
  MATLAB Function/1(u) -> u/1

== system Simulador_lineal/Sistema de control/PID roll ==
  setpoint : Inport
  sensor : Inport  Port=2
  sensorDerivada : Inport  Port=3
  habIntegral : Inport  Port=4
  tiempo : Inport  Port=5
  Constant : Constant  Value=Kp
  Constant1 : Constant  Value=Ki
  Constant2 : Constant  Value=Kd
  Constant3 : Constant  Value=Kff
  Constant4 : Constant  Value=LimI
  Constant5 : Constant  Value=LimT
  MATLAB Function : MATLAB Function  TreatAsAtomicUnit=on
  u : Outport
  wires:
  Constant/1 -> MATLAB Function/1(kp)
  Constant2/1 -> MATLAB Function/3(kd)
  habIntegral/1 -> MATLAB Function/10(habIntegral)
  Constant5/1 -> MATLAB Function/6(limTotal)
  Constant4/1 -> MATLAB Function/5(limIntegral)
  Constant3/1 -> MATLAB Function/4(kff)
  Constant1/1 -> MATLAB Function/2(ki)
  sensorDerivada/1 -> MATLAB Function/9(sensorDerivada)
  setpoint/1 -> MATLAB Function/7(setPoint)
  sensor/1 -> MATLAB Function/8(sensor)
  tiempo/1 -> MATLAB Function/11(tiempo)
  MATLAB Function/1(u) -> u/1

== system Simulador_lineal/Sistema de control/PID roll velocidad ==
  setpoint : Inport
  sensor : Inport  Port=2
  sensorDerivada : Inport  Port=3
  habIntegral : Inport  Port=4
  tiempo : Inport  Port=5
  Constant : Constant  Value=Kp
  Constant1 : Constant  Value=Ki
  Constant2 : Constant  Value=Kd
  Constant3 : Constant  Value=Kff
  Constant4 : Constant  Value=LimI
  Constant5 : Constant  Value=LimT
  MATLAB Function : MATLAB Function  TreatAsAtomicUnit=on
  u : Outport
  wires:
  MATLAB Function/1(u) -> u/1
  tiempo/1 -> MATLAB Function/11(tiempo)
  sensor/1 -> MATLAB Function/8(sensor)
  setpoint/1 -> MATLAB Function/7(setpoint)
  sensorDerivada/1 -> MATLAB Function/9(sensorDerivada)
  Constant1/1 -> MATLAB Function/2(ki)
  Constant3/1 -> MATLAB Function/4(kff)
  Constant4/1 -> MATLAB Function/5(limIntegral)
  Constant5/1 -> MATLAB Function/6(limTotal)
  habIntegral/1 -> MATLAB Function/10(habIntegral)
  Constant2/1 -> MATLAB Function/3(kd)
  Constant/1 -> MATLAB Function/1(kp)

== system Simulador_lineal/Sistema de control/PID yaw ==
  setpoint : Inport
  sensor : Inport  Port=2
  sensorDerivada : Inport  Port=3
  habIntegral : Inport  Port=4
  tiempo : Inport  Port=5
  Constant : Constant  Value=Kp
  Constant1 : Constant  Value=Ki
  Constant2 : Constant  Value=Kd
  Constant3 : Constant  Value=Kff
  Constant4 : Constant  Value=LimI
  Constant5 : Constant  Value=LimT
  MATLAB Function : MATLAB Function  TreatAsAtomicUnit=on
  u : Outport
  wires:
  MATLAB Function/1(u) -> u/1
  tiempo/1 -> MATLAB Function/11(tiempo)
  sensor/1 -> MATLAB Function/8(sensor)
  setpoint/1 -> MATLAB Function/7(setPoint)
  sensorDerivada/1 -> MATLAB Function/9(sensorDerivada)
  Constant1/1 -> MATLAB Function/2(ki)
  Constant3/1 -> MATLAB Function/4(kff)
  Constant4/1 -> MATLAB Function/5(limIntegral)
  Constant5/1 -> MATLAB Function/6(limTotal)
  habIntegral/1 -> MATLAB Function/10(habIntegral)
  Constant2/1 -> MATLAB Function/3(kd)
  Constant/1 -> MATLAB Function/1(kp)

== system Simulador_lineal/Sistema de control/PID yaw velocidad ==
  setpoint : Inport
  sensor : Inport  Port=2
  sensorDerivada : Inport  Port=3
  habIntegral : Inport  Port=4
  tiempo : Inport  Port=5
  Constant : Constant  Value=Kp
  Constant1 : Constant  Value=Ki
  Constant2 : Constant  Value=Kd
  Constant3 : Constant  Value=Kff
  Constant4 : Constant  Value=LimI
  Constant5 : Constant  Value=LimT
  MATLAB Function : MATLAB Function  TreatAsAtomicUnit=on
  u : Outport
  wires:
  Constant/1 -> MATLAB Function/1(kp)
  Constant2/1 -> MATLAB Function/3(kd)
  habIntegral/1 -> MATLAB Function/10(habIntegral)
  Constant5/1 -> MATLAB Function/6(limTotal)
  Constant4/1 -> MATLAB Function/5(limIntegral)
  Constant3/1 -> MATLAB Function/4(kff)
  Constant1/1 -> MATLAB Function/2(ki)
  sensorDerivada/1 -> MATLAB Function/9(sensorDerivada)
  setpoint/1 -> MATLAB Function/7(setPoint)
  sensor/1 -> MATLAB Function/8(sensor)
  tiempo/1 -> MATLAB Function/11(tiempo)
  MATLAB Function/1(u) -> u/1

== matlab function Simulador_lineal/Estimacion lineal/Filtro pasa bajos  acelerometro/MATLAB Function4 ==
  settings: updateMethod=DISCRETE
  data: In input; Fc input; Out output; Ts input
function Out  = LowPassFilterP1(In, Fc, Ts)

persistent b0 b1 a0 a1 in1 out1

if isempty(b0)
    ohm = 2.0 * pi * Fc;

    b1 = ohm * Ts;
    b0 = b1;
    a1 = 2.0 + b1;
    a0 = b1 - 2.0;

    in1  = 0;
    out1 = 0;
end

Out = (b1 * In + b0 * in1 - a0 * out1) / a1;

in1  = In;
out1 = Out;

== matlab function Simulador_lineal/Estimacion lineal/Filtro pasa bajos  acelerometro/MATLAB Function5 ==
  settings: updateMethod=DISCRETE
  data: In input; Fc input; Out output; Ts input
function Out  = LowPassFilterP2(In, Fc, Ts)

persistent b0 b1 b2 a1 a2 a0 in1 in2 out1 out2

if isempty(b0)
    ohm     = 2 * pi * Fc;
    damping = 1 / (sqrt(2));

    b2 = Ts^2 * ohm^2;
    b1 = 2.0 * b2;
    b0 = b2;

    a2 = 4.0 + 4.0 * damping * ohm * Ts + b2;
    a1 = -8.0 + b1;
    a0 = 4.0 - 4.0 * damping * ohm * Ts + b2;

    in1  = 0;
    in2  = 0;
    out1 = 0;
    out2 = 0;
end

Out = (b2 * In + b1 * in1 + b0 * in2 - a1 * out1 - a0 * out2) / a2;

in2  = in1;
in1  = In;
out2 = out1;
out1 = Out;

== matlab function Simulador_lineal/Estimacion lineal/Filtro pasa bajos  acelerometro/MATLAB Function6 ==
  settings: updateMethod=DISCRETE
  data: In input; Fc input; Out output; Ts input
function Out  = LowPassFilterP1(In, Fc, Ts)

persistent b0 b1 a0 a1 in1 out1

if isempty(b0)
    ohm = 2.0 * pi * Fc;

    b1 = ohm * Ts;
    b0 = b1;
    a1 = 2.0 + b1;
    a0 = b1 - 2.0;

    in1  = 0;
    out1 = 0;
end

Out = (b1 * In + b0 * in1 - a0 * out1) / a1;

in1  = In;
out1 = Out;

== matlab function Simulador_lineal/Sistema de control/MATLAB Function ==
  data: u input; pwm output size=4
function pwm = Mixer(u)
    pwm = [0 0 0 0]';
    
    pwm(1) = u(4) - u(1) + u(2) + u(3);
    pwm(2) = u(4) + u(1) + u(2) - u(3);
    pwm(3) = u(4) + u(1) - u(2) + u(3);   
    pwm(4) = u(4) - u(1) - u(2) - u(3);

== matlab function Simulador_lineal/Estimacion lineal/Filtro pasa bajos giroscopio/MATLAB Function1 ==
  settings: updateMethod=DISCRETE
  data: In input; Fc input; Out output; Ts input
function Out  = LowPassFilterP2(In, Fc, Ts)

persistent b0 b1 b2 a1 a2 a0 in1 in2 out1 out2

if isempty(b0)
    ohm     = 2 * pi * Fc;
    damping = 1 / (sqrt(2));

    b2 = Ts^2 * ohm^2;
    b1 = 2.0 * b2;
    b0 = b2;

    a2 = 4.0 + 4.0 * damping * ohm * Ts + b2;
    a1 = -8.0 + b1;
    a0 = 4.0 - 4.0 * damping * ohm * Ts + b2;

    in1  = 0;
    in2  = 0;
    out1 = 0;
    out2 = 0;
end

Out = (b2 * In + b1 * in1 + b0 * in2 - a1 * out1 - a0 * out2) / a2;

in2  = in1;
in1  = In;
out2 = out1;
out1 = Out;

== matlab function Simulador_lineal/Estimacion lineal/Filtro pasa bajos giroscopio/MATLAB Function2 ==
  settings: updateMethod=DISCRETE
  data: In input; Fc input; Out output; Ts input
function Out  = LowPassFilterP2(In, Fc, Ts)

persistent b0 b1 b2 a1 a2 a0 in1 in2 out1 out2

if isempty(b0)
    ohm     = 2 * pi * Fc;
    damping = 1 / (sqrt(2));

    b2 = Ts^2 * ohm^2;
    b1 = 2.0 * b2;
    b0 = b2;

    a2 = 4.0 + 4.0 * damping * ohm * Ts + b2;
    a1 = -8.0 + b1;
    a0 = 4.0 - 4.0 * damping * ohm * Ts + b2;

    in1  = 0;
    in2  = 0;
    out1 = 0;
    out2 = 0;
end

Out = (b2 * In + b1 * in1 + b0 * in2 - a1 * out1 - a0 * out2) / a2;

in2  = in1;
in1  = In;
out2 = out1;
out1 = Out;

== matlab function Simulador_lineal/Estimacion lineal/Filtro pasa bajos acel angular/MATLAB Function1 ==
  settings: updateMethod=DISCRETE
  data: In input; Fc input; Out output; Ts input
function Out  = LowPassFilterP2(In, Fc, Ts)

persistent b0 b1 b2 a1 a2 a0 in1 in2 out1 out2

if isempty(b0)
    ohm     = 2 * pi * Fc;
    damping = 1 / (sqrt(2));

    b2 = Ts^2 * ohm^2;
    b1 = 2.0 * b2;
    b0 = b2;

    a2 = 4.0 + 4.0 * damping * ohm * Ts + b2;
    a1 = -8.0 + b1;
    a0 = 4.0 - 4.0 * damping * ohm * Ts + b2;

    in1  = 0;
    in2  = 0;
    out1 = 0;
    out2 = 0;
end

Out = (b2 * In + b1 * in1 + b0 * in2 - a1 * out1 - a0 * out2) / a2;

in2  = in1;
in1  = In;
out2 = out1;
out1 = Out;

== matlab function Simulador_lineal/Estimacion lineal/Filtro pasa bajos acel angular/MATLAB Function2 ==
  settings: updateMethod=DISCRETE
  data: In input; Fc input; Out output; Ts input
function Out  = LowPassFilterP2(In, Fc, Ts)

persistent b0 b1 b2 a1 a2 a0 in1 in2 out1 out2

if isempty(b0)
    ohm     = 2 * pi * Fc;
    damping = 1 / (sqrt(2));

    b2 = Ts^2 * ohm^2;
    b1 = 2.0 * b2;
    b0 = b2;

    a2 = 4.0 + 4.0 * damping * ohm * Ts + b2;
    a1 = -8.0 + b1;
    a0 = 4.0 - 4.0 * damping * ohm * Ts + b2;

    in1  = 0;
    in2  = 0;
    out1 = 0;
    out2 = 0;
end

Out = (b2 * In + b1 * in1 + b0 * in2 - a1 * out1 - a0 * out2) / a2;

in2  = in1;
in1  = In;
out2 = out1;
out1 = Out;

== matlab function Simulador_lineal/Estimacion lineal/Filtro pasa bajos acel angular/MATLAB Function3 ==
  settings: updateMethod=DISCRETE
  data: In input; Fc input; Out output; Ts input
function Out  = LowPassFilterP1(In, Fc, Ts)

persistent b0 b1 a0 a1 in1 out1

if isempty(b0)
    ohm = 2.0 * pi * Fc;

    b1 = ohm * Ts;
    b0 = b1;
    a1 = 2.0 + b1;
    a0 = b1 - 2.0;

    in1  = 0;
    out1 = 0;
end

Out = (b1 * In + b0 * in1 - a0 * out1) / a1;

in1  = In;
out1 = Out;

== matlab function Simulador_lineal/Estimacion lineal/Filtro pasa bajos acel angular/MATLAB Function4 ==
  settings: updateMethod=DISCRETE
  data: In input; Fc input; Out output; Ts input
function Out  = LowPassFilterP1(In, Fc, Ts)

persistent b0 b1 a0 a1 in1 out1

if isempty(b0)
    ohm = 2.0 * pi * Fc;

    b1 = ohm * Ts;
    b0 = b1;
    a1 = 2.0 + b1;
    a0 = b1 - 2.0;

    in1  = 0;
    out1 = 0;
end

Out = (b1 * In + b0 * in1 - a0 * out1) / a1;

in1  = In;
out1 = Out;

== matlab function Simulador_lineal/Estimacion lineal/Filtro pasa bajos acel angular/MATLAB Function5 ==
  settings: updateMethod=DISCRETE
  data: In input; Fc input; Out output; Ts input
function Out  = LowPassFilterP2(In, Fc, Ts)

persistent b0 b1 b2 a1 a2 a0 in1 in2 out1 out2

if isempty(b0)
    ohm     = 2 * pi * Fc;
    damping = 1 / (sqrt(2));

    b2 = Ts^2 * ohm^2;
    b1 = 2.0 * b2;
    b0 = b2;

    a2 = 4.0 + 4.0 * damping * ohm * Ts + b2;
    a1 = -8.0 + b1;
    a0 = 4.0 - 4.0 * damping * ohm * Ts + b2;

    in1  = 0;
    in2  = 0;
    out1 = 0;
    out2 = 0;
end

Out = (b2 * In + b1 * in1 + b0 * in2 - a1 * out1 - a0 * out2) / a2;

in2  = in1;
in1  = In;
out2 = out1;
out1 = Out;

== matlab function Simulador_lineal/Estimacion lineal/Filtro pasa bajos acel angular/MATLAB Function6 ==
  settings: updateMethod=DISCRETE
  data: In input; Fc input; Out output; Ts input
function Out  = LowPassFilterP1(In, Fc, Ts)

persistent b0 b1 a0 a1 in1 out1

if isempty(b0)
    ohm = 2.0 * pi * Fc;

    b1 = ohm * Ts;
    b0 = b1;
    a1 = 2.0 + b1;
    a0 = b1 - 2.0;

    in1  = 0;
    out1 = 0;
end

Out = (b1 * In + b0 * in1 - a0 * out1) / a1;

in1  = In;
out1 = Out;

== matlab function Simulador_lineal/Estimacion lineal/Filtro pasa bajos giroscopio/MATLAB Function3 ==
  settings: updateMethod=DISCRETE
  data: In input; Fc input; Out output; Ts input
function Out  = LowPassFilterP1(In, Fc, Ts)

persistent b0 b1 a0 a1 in1 out1

if isempty(b0)
    ohm = 2.0 * pi * Fc;

    b1 = ohm * Ts;
    b0 = b1;
    a1 = 2.0 + b1;
    a0 = b1 - 2.0;

    in1  = 0;
    out1 = 0;
end

Out = (b1 * In + b0 * in1 - a0 * out1) / a1;

in1  = In;
out1 = Out;

== matlab function Simulador_lineal/Estimacion lineal/Filtro pasa bajos giroscopio/MATLAB Function4 ==
  settings: updateMethod=DISCRETE
  data: In input; Fc input; Out output; Ts input
function Out  = LowPassFilterP1(In, Fc, Ts)

persistent b0 b1 a0 a1 in1 out1

if isempty(b0)
    ohm = 2.0 * pi * Fc;

    b1 = ohm * Ts;
    b0 = b1;
    a1 = 2.0 + b1;
    a0 = b1 - 2.0;

    in1  = 0;
    out1 = 0;
end

Out = (b1 * In + b0 * in1 - a0 * out1) / a1;

in1  = In;
out1 = Out;

== matlab function Simulador_lineal/Estimacion lineal/Filtro pasa bajos giroscopio/MATLAB Function5 ==
  settings: updateMethod=DISCRETE
  data: In input; Fc input; Out output; Ts input
function Out  = LowPassFilterP2(In, Fc, Ts)

persistent b0 b1 b2 a1 a2 a0 in1 in2 out1 out2

if isempty(b0)
    ohm     = 2 * pi * Fc;
    damping = 1 / (sqrt(2));

    b2 = Ts^2 * ohm^2;
    b1 = 2.0 * b2;
    b0 = b2;

    a2 = 4.0 + 4.0 * damping * ohm * Ts + b2;
    a1 = -8.0 + b1;
    a0 = 4.0 - 4.0 * damping * ohm * Ts + b2;

    in1  = 0;
    in2  = 0;
    out1 = 0;
    out2 = 0;
end

Out = (b2 * In + b1 * in1 + b0 * in2 - a1 * out1 - a0 * out2) / a2;

in2  = in1;
in1  = In;
out2 = out1;
out1 = Out;

== matlab function Simulador_lineal/Estimacion lineal/Filtro pasa bajos giroscopio/MATLAB Function6 ==
  settings: updateMethod=DISCRETE
  data: In input; Fc input; Out output; Ts input
function Out  = LowPassFilterP1(In, Fc, Ts)

persistent b0 b1 a0 a1 in1 out1

if isempty(b0)
    ohm = 2.0 * pi * Fc;

    b1 = ohm * Ts;
    b0 = b1;
    a1 = 2.0 + b1;
    a0 = b1 - 2.0;

    in1  = 0;
    out1 = 0;
end

Out = (b1 * In + b0 * in1 - a0 * out1) / a1;

in1  = In;
out1 = Out;

== matlab function Simulador_lineal/Sistema de control/PID pitch/MATLAB Function ==
  data: kp input; u output; ki input; kd input; kff input; limIntegral input; limTotal input; setPoint input; sensor input; sensorDerivada input; habIntegral input; tiempo input
function u = ControlPID(kp, ki, kd, kff, limIntegral, limTotal, setPoint, sensor, sensorDerivada, habIntegral, tiempo)

persistent integral tiempoAnterior

if isempty(integral)
    integral = 0;
    tiempoAnterior = 0;
end

dt = tiempo - tiempoAnterior;
tiempoAnterior = tiempo;

error  = setPoint - sensor;
salida = error * kp + ki - sensorDerivada * kd + setPoint * kff;

if habIntegral 
    integral = integral + error * dt * ki;

    if integral > limIntegral
        integral = limIntegral;
    elseif integral < -limIntegral
        integral = -limIntegral;
    end
end

if salida > limTotal
    salida = limTotal;
elseif salida < -limTotal
    salida = -limTotal;
end

u = salida;

== matlab function Simulador_lineal/Sistema de control/PID roll/MATLAB Function ==
  data: kp input; u output; ki input; kd input; kff input; limIntegral input; limTotal input; setPoint input; sensor input; sensorDerivada input; habIntegral input; tiempo input
function u = ControlPID(kp, ki, kd, kff, limIntegral, limTotal, setPoint, sensor, sensorDerivada, habIntegral, tiempo)

persistent integral tiempoAnterior

if isempty(integral)
    integral = 0;
    tiempoAnterior = 0;
end

dt = tiempo - tiempoAnterior;
tiempoAnterior = tiempo;

error  = setPoint - sensor;
salida = error * kp + ki - sensorDerivada * kd + setPoint * kff;

if habIntegral 
    integral = integral + error * dt * ki;

    if integral > limIntegral
        integral = limIntegral;
    elseif integral < -limIntegral
        integral = -limIntegral;
    end
end

if salida > limTotal
    salida = limTotal;
elseif salida < -limTotal
    salida = -limTotal;
end

u = salida;

== matlab function Simulador_lineal/Sistema de control/PID yaw/MATLAB Function ==
  data: kp input; u output; ki input; kd input; kff input; limIntegral input; limTotal input; setPoint input; sensor input; sensorDerivada input; habIntegral input; tiempo input
function u = ControlPID(kp, ki, kd, kff, limIntegral, limTotal, setPoint, sensor, sensorDerivada, habIntegral, tiempo)

persistent integral tiempoAnterior

if isempty(integral)
    integral = 0;
    tiempoAnterior = 0;
end

dt = tiempo - tiempoAnterior;
tiempoAnterior = tiempo;

error  = setPoint - sensor;
salida = error * kp + ki - sensorDerivada * kd + setPoint * kff;

if habIntegral 
    integral = integral + error * dt * ki;

    if integral > limIntegral
        integral = limIntegral;
    elseif integral < -limIntegral
        integral = -limIntegral;
    end
end

if salida > limTotal
    salida = limTotal;
elseif salida < -limTotal
    salida = -limTotal;
end

u = salida;

== matlab function Simulador_lineal/Sistema de control/PID pitch velocidad/MATLAB Function ==
  data: kp input; u output; ki input; kd input; kff input; limIntegral input; limTotal input; setPoint input; sensor input; sensorDerivada input; habIntegral input; tiempo input
function u = ControlPID(kp, ki, kd, kff, limIntegral, limTotal, setPoint, sensor, sensorDerivada, habIntegral, tiempo)

persistent integral tiempoAnterior

if isempty(integral)
    integral = 0;
    tiempoAnterior = 0;
end

dt = tiempo - tiempoAnterior;
tiempoAnterior = tiempo;

error  = setPoint - sensor;
salida = error * kp + ki - sensorDerivada * kd + setPoint * kff;

if habIntegral 
    integral = integral + error * dt * ki;

    if integral > limIntegral
        integral = limIntegral;
    elseif integral < -limIntegral
        integral = -limIntegral;
    end
end

if salida > limTotal
    salida = limTotal;
elseif salida < -limTotal
    salida = -limTotal;
end

u = salida;

== matlab function Simulador_lineal/Sistema de control/PID roll velocidad/MATLAB Function ==
  data: kp input; u output; ki input; kd input; kff input; limIntegral input; limTotal input; setpoint input; sensor input; sensorDerivada input; habIntegral input; tiempo input
function u = ControlPID(kp, ki, kd, kff, limIntegral, limTotal, setpoint, sensor, sensorDerivada, habIntegral, tiempo)

persistent integral tiempoAnterior

if isempty(integral)
    integral = 0;
    tiempoAnterior = 0;
end

dt = tiempo - tiempoAnterior;
tiempoAnterior = tiempo;

error  = setpoint - sensor;
salida = error * kp + ki - sensorDerivada * kd + setpoint * kff;

if habIntegral 
    integral = integral + error * dt * ki;

    if integral > limIntegral
        integral = limIntegral;
    elseif integral < -limIntegral
        integral = -limIntegral;
    end
end

if salida > limTotal
    salida = limTotal;
elseif salida < -limTotal
    salida = -limTotal;
end

u = salida;

== matlab function Simulador_lineal/Sistema de control/PID yaw velocidad/MATLAB Function ==
  data: kp input; u output; ki input; kd input; kff input; limIntegral input; limTotal input; setPoint input; sensor input; sensorDerivada input; habIntegral input; tiempo input
function u = ControlPID(kp, ki, kd, kff, limIntegral, limTotal, setPoint, sensor, sensorDerivada, habIntegral, tiempo)

persistent integral tiempoAnterior

if isempty(integral)
    integral = 0;
    tiempoAnterior = 0;
end

dt = tiempo - tiempoAnterior;
tiempoAnterior = tiempo;

error  = setPoint - sensor;
salida = error * kp + ki - sensorDerivada * kd + setPoint * kff;

if habIntegral 
    integral = integral + error * dt * ki;

    if integral > limIntegral
        integral = limIntegral;
    elseif integral < -limIntegral
        integral = -limIntegral;
    end
end

if salida > limTotal
    salida = limTotal;
elseif salida < -limTotal
    salida = -limTotal;
end

u = salida;

== matlab function Simulador_lineal/Sistema de control/MATLAB Function2 ==
  data: Euler input; Wb output; Vel input
function Wb = RotacionVelTB(Euler, Vel)

w = [0 0 0]';

w(1) = Vel(1) - sin(Euler(2)) * Vel(3);
w(2) = cos(Euler(1)) * Vel(2)   + sin(Euler(1)) * cos(Euler(2)) * Vel(3);
w(3) = - sin(Euler(1)) * Vel(2) + cos(Euler(2)) * cos(Euler(1)) * Vel(3);

Wb = w;

== matlab function Simulador_lineal/Modelo UAV lineal/Dinamica UAV/Modelo ==
  settings: updateMethod=DISCRETE
  data: Ab output; T input; Delta input; Gb output; I input; Im input; B input; F input; dM input; M input; Dr input; Dp input; Mo input; HabYaw input; HabAcel input; Wb input size=3; Velb input size=3; Q input size=4; Tiempo input; Al output
  function [Ab, Gb, Al] = Modelo(T, Delta, I,Im, B, F, dM, M, Dr, Dp, Mo, HabYaw, HabAcel, Wb, Velb, Q, Tiempo)
% Modelo matemático del UAV 

%%%%%%%%%%%%%%%%%%%%%%%%%%%%%%% ENTRADAS %%%%%%%%%%%%%%%%%%%%%%%%%%%%%%%%%%%%%%%%%%%%%%%%%%
% T     -> Fuerza de sustentación
% Delta -> Par de arraste 
% Wm    -> Velocidad de rotacion de los rotores
% I     -> Inercia del dron
% Im    -> Inercia del rotor
% B     -> Friccion viscosa
% F     -> Friccion estatica
% dM    -> Distancia al centro de masas
% M     -> Masa del dron
% Dr    -> Distancia al eje roll
% Dp    -> Distancia al eje pitch
% Mo    -> Par inicial
% HabYaw -> Habilitacion de yaw
% HabAcel
% Wb    -> Velocidades angulares en el cuerpo
% Euler -> Angulos de Euler


%%%%%%%%%%%%%%%%%%%%%%%%%%%%%%% SALIDAS %%%%%%%%%%%%%%%%%%%%%%%%%%%%%%%%%%%%%%%%%%%%%%%%%%%
% Ab  -> Aceleración angular en los 3 ejes
% Gb  -> Gravedad en el sistema de referencia del dron


%%%%%%%%%%%%%%%%%%%%%%%%%%%%% CONSTANTES %%%%%%%%%%%%%%%%%%%%%%%%%%%%%%%%%%%%%%%%%%%%%%%%%%
persistent g LrAnt TiempoAnterior

if isempty(g)
    g = 9.81;
    LrAnt = 0;
    TiempoAnterior = 0;
end


%%%%%%%%%%%%%%%%%%%%%%%%%%%%%% VARIABLES %%%%%%%%%%%%%%%%%%%%%%%%%%%%%%%%%%%%%%%%%%%%%%%%%%
Fe = zeros(1,3);
Euler = zeros(1,3);

dt = Tiempo - TiempoAnterior;
TiempoAnterior = Tiempo;


%%%%%%%%%%%%%%%%%%%%%%%%% ANGULOS Y ROTACIONES %%%%%%%%%%%%%%%%%%%%%%%%%%%%%%%%%%%%%%%%%%%%
% Angulos de Euler
Euler(1) = atan2(2 * Q(3) * Q(4) + 2 * Q(1) * Q(2), 2 * Q(1) * Q(1) + 2 * Q(4) * Q(4) - 1);
Euler(2) = -asin(2 * (Q(2) * Q(4) - Q(1) * Q(3)));
Euler(3) = atan2(2 * Q(2) * Q(3) + 2 * Q(1) * Q(4), 2 * Q(1) * Q(1) + 2 * Q(2) * Q(2) - 1);

% Matriz de rotación
R = [[1-2*Q(3)^2-2*Q(4)^2 2*(Q(2)*Q(3)+Q(1)*Q(4)) 2*(Q(2)*Q(4)-Q(1)*Q(3))];...
    [2*(Q(2)*Q(3)-Q(1)*Q(4)) 1-2*Q(2)^2-2*Q(4)^2 2*(Q(3)*Q(4)+Q(1)*Q(2))];...
    [2*(Q(2)*Q(4)+Q(1)*Q(3)) 2*(Q(3)*Q(4)-Q(1)*Q(2)) 1-2*Q(2)^2-2*Q(3)^2]];


%%%%%%%%%%%%%%%%%%%%%%%%%%% DINAMICA ANGULAR %%%%%%%%%%%%%%%%%%%%%%%%%%%%%%%%%%%%%%%%%%%%%%
% Pares generados por los rotores
Mx = Dr * (T(2) + T(3) - T(1) - T(4));              
My = Dp * (T(1) + T(2) - T(3) - T(4));               
Mz = Delta(1) - Delta(2) + Delta(3) - Delta(4); 

% Calculo de inercia de la masa rotante de los motores
%Lr  = Im * (- Wm(1) + Wm(2) - Wm(3) + Wm(4));
%ALr = (Lr - LrAnt) / dt;
%LrAnt = Lr;

% Fricción estatica
Fe(1) = sign(Wb(1)) * F(1);
Fe(2) = sign(Wb(2)) * F(2);
Fe(3) = sign(Wb(3)) * F(3);

% Momentos en la aeronave
Tx = Mx; % + (I(2) - I(3)) * Wb(2) * Wb(3) - Lr * Wb(2) - B(1) * Wb(1) - Fe(1) + Mo(1) - M * g * dM * sin(Euler(1));
Ty = My; % + (I(3) - I(1)) * Wb(1) * Wb(3) - Lr * Wb(1) - B(2) * Wb(2) - Fe(2) + Mo(2) - M * g * dM * cos(Euler(1)) * sin(Euler(2));

if HabYaw
    Tz = Mz; % + Wb(1) * I(1) * 2 + Wb(2) * I(2) + ALr  - B(3) * Wb(3) - Fe(3) + Mo(3);
else
    Tz = 0;
end

% Obtención de la aceleracion angular
Ax = Tx / I(1);
Ay = Ty / I(2);
Az = Tz / I(3);

Ab = [Ax Ay Az]';


%%%%%%%%%%%%%%%%%%%%%%%%%%% DINAMICA LINEAL %%%%%%%%%%%%%%%%%%%%%%%%%%%%%%%%%%%%%%%%%%%%%%%
% Gravedad con respecto al body
Gb = R * [0 0 1]';

% Aceleraciones lineales
if HabAcel
    AcelX = Gb(1) * g + Wb(3) * Velb(2) - Wb(2) * Velb(3);                                                 
    AcelY = Gb(2) * g + Wb(1) * Velb(3) - Wb(3) * Velb(1);                                                 
    AcelZ = Gb(3) * g + Wb(2) * Velb(1) - Wb(1) * Velb(2) - (T(1) + T(2) + T(3) + T(4)) / M;
    
    Al = [AcelX AcelY AcelZ]';
else
    Al = [0 0 0]';
end

== matlab function Simulador_lineal/Modelo UAV lineal/Dinamica UAV/Rotacion ==
  settings: updateMethod=DISCRETE
  data: Q output; Wb input size=3; Euler output size=3; Tiempo input
function [Q, Euler] = RotacionAngular(Wb, Tiempo)

persistent q TiempoAnterior

if isempty(q)
    q  = [1 0 0 0];
    TiempoAnterior = 0;
end

dt = Tiempo - TiempoAnterior;
TiempoAnterior = Tiempo;

W = [0 0 0]';
Euler = [0 0 0]';

% Se integra la tasa de cambio de cuaternion
W(1) = Wb(1) * (0.5 * dt);
W(2) = Wb(2) * (0.5 * dt);
W(3) = Wb(3) * (0.5 * dt);

q1 = q(1);
q2 = q(2);
q3 = q(3);

q(1) = q(1) + (-q2 * W(1) - q3 * W(2) - q(4) * W(3));
q(2) = q(2) + ( q1 * W(1) + q3 * W(3) - q(4) * W(2));
q(3) = q(3) + ( q1 * W(2) - q2 * W(3) + q(4) * W(1));
q(4) = q(4) + ( q1 * W(3) + q2 * W(2) - q3   * W(1));


% Se normaliza el cuaternion
Q = q / norm(q);

% Ecuaciones sacadas de Madgwick con el conjugado implicito en las formulas
Euler(1) = atan2(2 * Q(3) * Q(4) + 2 * Q(1) * Q(2), 2 * Q(1) * Q(1) + 2 * Q(4) * Q(4) - 1);
Euler(2) = -asin(2 * (Q(2) * Q(4) - Q(1) * Q(3)));
Euler(3) = atan2(2 * Q(2) * Q(3) + 2 * Q(1) * Q(4), 2 * Q(1) * Q(1) + 2 * Q(2) * Q(2) - 1);

== matlab function Simulador_lineal/Estimacion lineal/Filtro pasa bajos  acelerometro/MATLAB Function1 ==
  settings: updateMethod=DISCRETE
  data: In input; Fc input; Out output; Ts input
function Out  = LowPassFilterP2(In, Fc, Ts)

persistent b0 b1 b2 a1 a2 a0 in1 in2 out1 out2

if isempty(b0)
    ohm     = 2 * pi * Fc;
    damping = 1 / (sqrt(2));

    b2 = Ts^2 * ohm^2;
    b1 = 2.0 * b2;
    b0 = b2;

    a2 = 4.0 + 4.0 * damping * ohm * Ts + b2;
    a1 = -8.0 + b1;
    a0 = 4.0 - 4.0 * damping * ohm * Ts + b2;

    in1  = 0;
    in2  = 0;
    out1 = 0;
    out2 = 0;
end

Out = (b2 * In + b1 * in1 + b0 * in2 - a1 * out1 - a0 * out2) / a2;

in2  = in1;
in1  = In;
out2 = out1;
out1 = Out;

== matlab function Simulador_lineal/Estimacion lineal/Filtro pasa bajos  acelerometro/MATLAB Function2 ==
  settings: updateMethod=DISCRETE
  data: In input; Fc input; Out output; Ts input
function Out  = LowPassFilterP2(In, Fc, Ts)

persistent b0 b1 b2 a1 a2 a0 in1 in2 out1 out2

if isempty(b0)
    ohm     = 2 * pi * Fc;
    damping = 1 / (sqrt(2));

    b2 = Ts^2 * ohm^2;
    b1 = 2.0 * b2;
    b0 = b2;

    a2 = 4.0 + 4.0 * damping * ohm * Ts + b2;
    a1 = -8.0 + b1;
    a0 = 4.0 - 4.0 * damping * ohm * Ts + b2;

    in1  = 0;
    in2  = 0;
    out1 = 0;
    out2 = 0;
end

Out = (b2 * In + b1 * in1 + b0 * in2 - a1 * out1 - a0 * out2) / a2;

in2  = in1;
in1  = In;
out2 = out1;
out1 = Out;

== matlab function Simulador_lineal/Estimacion lineal/Filtro pasa bajos  acelerometro/MATLAB Function3 ==
  settings: updateMethod=DISCRETE
  data: In input; Fc input; Out output; Ts input
function Out  = LowPassFilterP1(In, Fc, Ts)

persistent b0 b1 a0 a1 in1 out1

if isempty(b0)
    ohm = 2.0 * pi * Fc;

    b1 = ohm * Ts;
    b0 = b1;
    a1 = 2.0 + b1;
    a0 = b1 - 2.0;

    in1  = 0;
    out1 = 0;
end

Out = (b1 * In + b0 * in1 - a0 * out1) / a1;

in1  = In;
out1 = Out;
